simulink model "Blocks_LQR"  (R2020a)
settings: Solver=VariableStepAuto  StartTime=0.0  StopTime=50  RelTol=1e-3
values from neighbouring files (symbols this model uses):
  A = [0,-20,10]    [Animation_Obstacles.m]    (also in Blocks_LQR.m = [0 0 0 0 0 0 1 0 0 0 0 0; Blocks_LQRbasic.m = [0,1;-30,-1]; MPC.m = [a [0;0;0]; c*a 1 ]; animation_LQR.m = [-6,-10,-7])
  B = [0,-22,10]    [Animation_Obstacles.m]    (also in Blocks_LQR.m = [0 0 0 0; Blocks_LQRbasic.m = [0;2]; MPC.m = [b;c*b]; animation_LQR.m = [-6,-11,-7])
  C = [0,-22,-10]    [Animation_Obstacles.m]    (also in Blocks_LQR.m = diag([1,1,1,1,1,1,1,1,1,1,1,1]); Blocks_LQRbasic.m = [1,0]; MPC.m = [0 0 0 1]; animation_LQR.m = [-6,-11,-9])
  L = 2.75E-6    (= 2.75e-06)    [MPC.m]
  x0 = zeros(12,1)    [Blocks_LQR.m]    (also in LQGControl.m; LQRControl.m; LQRcontrol_with_Integrator.m; animation_LQG.m = 10)
undefined symbols (not defined in the file or in its folder): Kx, Kz
settings Model: Creator=Xrisostomos  LastModifiedBy=xriso

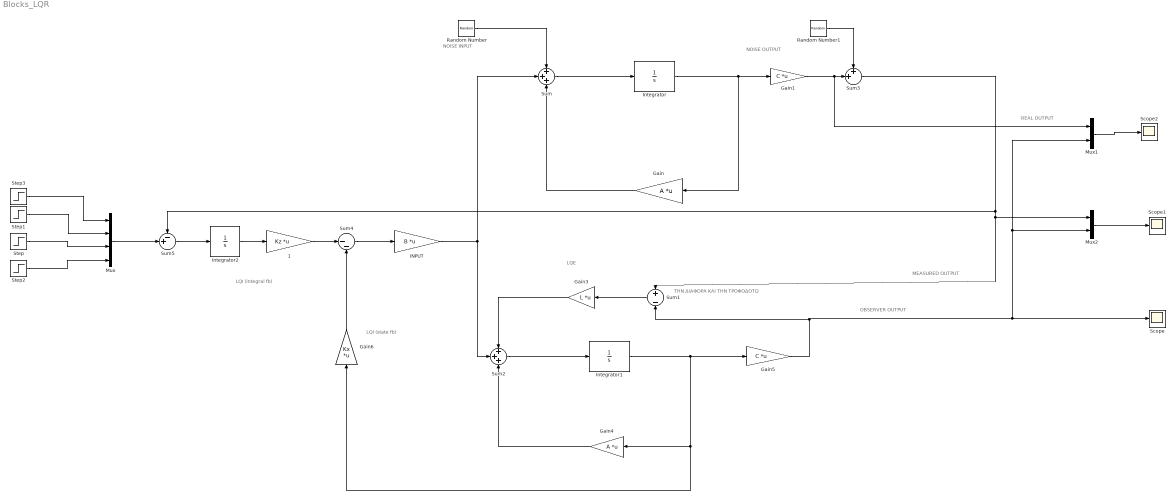
== system Blocks_LQR ==
  note: ΤΗΝ ΔΙΑΦΟΡΑ ΚΑΙ ΤΗΝ ΤΡΟΦΟΔΟΤΩ
  note: LQE
  note: OBSERVER OUTPUT
  note: MEASURED OUTPUT
  note: REAL OUTPUT
  note: NOISE OUTPUT
  note: NOISE INPUT
  note: LQI
      | (state fb)
  note: LQI
      | (integral fb)
  1 : Gain  Gain=Kz  Multiplication=Matrix(K*u)
  Gain : Gain  Gain=A  Multiplication=Matrix(K*u)
  Gain1 : Gain  Gain=C  Multiplication=Matrix(K*u)
  Gain3 : Gain  Gain=L  Multiplication=Matrix(K*u)
  Gain4 : Gain  Gain=A  Multiplication=Matrix(K*u)
  Gain5 : Gain  Gain=C  Multiplication=Matrix(K*u)
  Gain6 : Gain  Gain=Kx  Multiplication=Matrix(K*u)
  INPUT : Gain  Gain=B  Multiplication=Matrix(K*u)
  Integrator : Integrator  InitialCondition=x0
  Integrator1 : Integrator  InitialCondition=x0
  Integrator2 : Integrator  InitialCondition=x0
  Mux : Mux
  Mux1 : Mux  Inputs=2
  Mux2 : Mux  Inputs=2
  Random Number : RandomNumber  SampleTime=0.1
  Random Number1 : RandomNumber  SampleTime=0.1
  Scope : Scope
  Scope1 : Scope
  Scope2 : Scope
  Step{,1..3} (4 alike) : Step  SampleTime=0
  Sum : Sum  Inputs=+++
  Sum1 : Sum  Inputs=+-
  Sum2 : Sum  Inputs=+++
  Sum3 : Sum  Inputs=++|
  Sum4 : Sum  Inputs=|--
  Sum5 : Sum  Inputs=-+|
  wires:
  Sum/1 -> Integrator/1
  Integrator/1 -> Gain1/1, Gain/1
  INPUT/1 -> Sum/2, Sum2/2
  Sum1/1 -> Gain3/1
  Gain1/1 -> Mux1/1, Sum3/2
  Gain3/1 -> Sum2/1
  Sum2/1 -> Integrator1/1
  Gain4/1 -> Sum2/3
  Integrator1/1 -> Gain6/1, Gain4/1, Gain5/1
  Gain5/1 -> Sum1/2, Mux1/2, Mux2/2, Scope/1
  Step1/1 -> Mux/2
  Gain/1 -> Sum/3
  Random Number/1 -> Sum/1
  Sum3/1 -> Sum5/1, Mux2/1, Sum1/1
  Random Number1/1 -> Sum3/1
  Mux1/1 -> Scope2/1
  Mux2/1 -> Scope1/1
  Step3/1 -> Mux/1
  Gain6/1 -> Sum4/2
  Sum4/1 -> INPUT/1
  Step/1 -> Mux/3
  Step2/1 -> Mux/4
  Mux/1 -> Sum5/2
  Sum5/1 -> Integrator2/1
  1/1 -> Sum4/1
  Integrator2/1 -> 1/1
